simulink model "renew_energy_assignment1_t2andt3"  (R2024b)
settings: Solver=VariableStepAuto  StartTime=0.0  StopTime=100  RelTol=1e-3
values from neighbouring files (symbols this model uses):
  Tr = Tr_values(i)    [parameters_asign1_part2.m]    (also in parameters_asign1_t2andt3.m)
libraries: simulink x1
settings Model: Creator=zeyneptutumlu  LastModifiedBy=X13-G2JL
settings DataIOCC: SaveOutput=off  SaveTime=off
settings ModelReferenceCC: UpdateModelReferenceTargets=IfOutOfDate

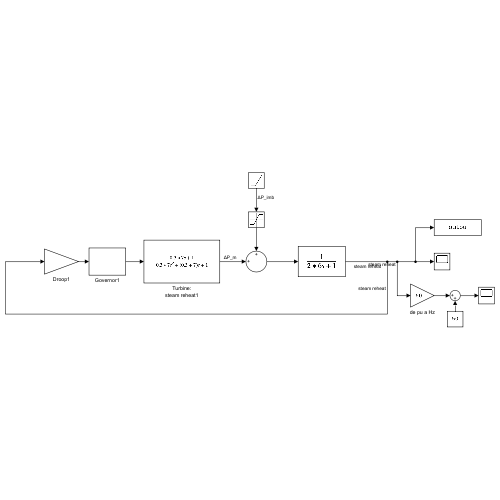
[thumbnail: Simulink's stored preview of the top-level diagram]
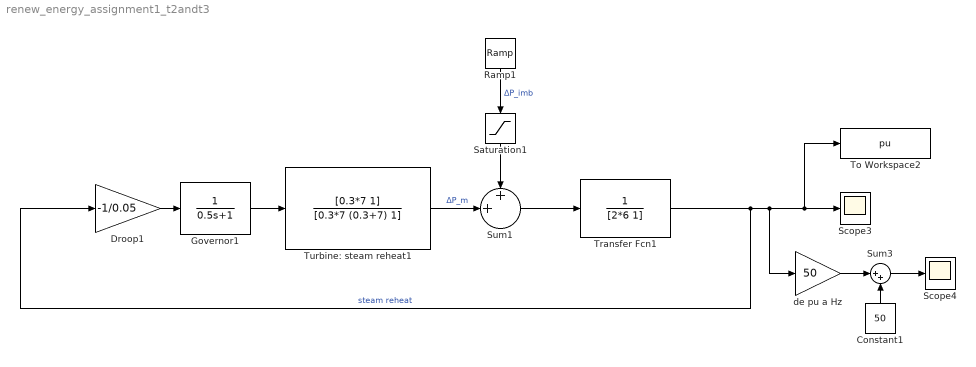
== system renew_energy_assignment1_t2andt3 ==
  Constant1 : Constant  Value=50
  Droop1 : Gain  Gain=-1/0.05
  Governor1 : TransferFcn  Denominator=[0.5 1]
  Ramp1 : simulink/Sources/Ramp  slope=-0.1/Tr  start=0  InitialOutput=0
  Saturation1 : Saturate  UpperLimit=0  LowerLimit=-0.1
  Scope3 : Scope
  Scope4 : Scope
  Sum1 : Sum  Inputs=++|
  Sum3 : Sum  Inputs=|++
  To Workspace2 : ToWorkspace  VariableName=pu  SaveFormat=Structure With Time  SampleTime=-1
  Transfer Fcn1 : TransferFcn  Denominator=[2*6 1]
  Turbine: steam reheat1 : TransferFcn  Numerator=[0.3*7 1]  Denominator=[0.3*7 (0.3+7) 1]
  de pu a Hz : Gain  Gain=50
  wires:
  Droop1/1 -> Governor1/1
  Saturation1/1 -> Sum1/1
  Turbine: steam reheat1/1 -> Sum1/2  "ΔP_m"
  Ramp1/1 -> Saturation1/1  "ΔP_imb"
  Governor1/1 -> Turbine: steam reheat1/1
  Sum1/1 -> Transfer Fcn1/1
  Transfer Fcn1/1 -> Droop1/1, de pu a Hz/1, To Workspace2/1, Scope3/1  "steam reheat"
  de pu a Hz/1 -> Sum3/1
  Constant1/1 -> Sum3/2
  Sum3/1 -> Scope4/1
